simulink model "cruise_model_open_loop"  (R2017a)
settings: Solver=VariableStepAuto  StartTime=0.0  StopTime=700  RelTol=1e-3
settings Model: Creator=root  LastModifiedBy=root

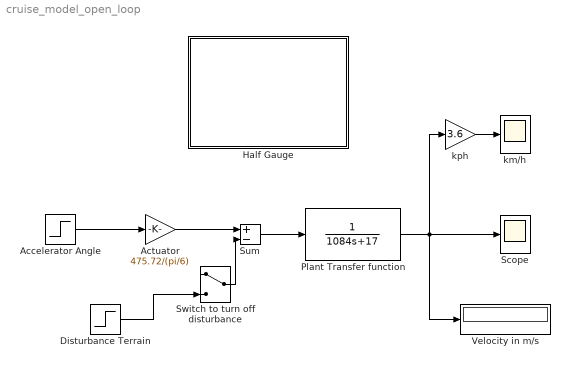
== system cruise_model_open_loop ==
  Accelerator Angle : Step  After=pi/6  SampleTime=0
  Actuator : Gain  Gain=475.72/(pi/6)
  Disturbance Terrain : Step  Time=350  After=475.72*9.81*sin(pi/45)  SampleTime=0
  Half Gauge : Subsystem  DialogController=hmiCreateDDGDialog  IsWebBlock=on  mask(MWDashboardBlock){webBlockId=c77fd51c-fd22-40a0-8bec-fa9513db74d2, webBlockType=semicirculargauge, ShowInLibBrowser=on, ShowInitialText=on, HMISrcModelName=cruise_model_open_loop}
      mask prompts: webBlockId "WebBlock Id"; webBlockType "WebBlock Type"; HMISrcModelName "Source Model"
      mask help: SimulinkHMI:dialogs:SemicircularGaugeDialogDesc
      mask Help: helpview([docroot '/mapfiles/simulink.map'], 'hmi_half_gauge')
      mask Display:
      | if strcmp(get_param(bdroot(gcb),'BlockDiagramType'), 'library')
      |     image([(matlabroot) '/toolbox/simulink/hmi/icons/SemicircularGauge.png']);
      | end
  Plant Transfer function : TransferFcn  Denominator=[1084 17]
  Scope : Scope
  Sum : Sum  Inputs=+-
  Switch to turn off disturbance : ManualSwitch
  Velocity in m/s : Display
  km/h : Scope
  kph : Gain  Gain=3.6
  wires:
  Accelerator Angle/1 -> Actuator/1
  Plant Transfer function/1 -> Velocity in m/s/1, kph/1, Scope/1
  kph/1 -> km/h/1
  Actuator/1 -> Sum/1
  Sum/1 -> Plant Transfer function/1
  Disturbance Terrain/1 -> Switch to turn off disturbance/2
  Switch to turn off disturbance/1 -> Sum/2

== system cruise_model_open_loop/Half Gauge ==
